simulink subsystem "SubsystemT"  (R2021a)
settings: Solver=VariableStepAuto  StartTime=0.0  StopTime=10.0  RelTol=1e-3
libraries: dspmathops x1, sharedtransform x1
settings Model: Creator=noraw  LastModifiedBy=noraw

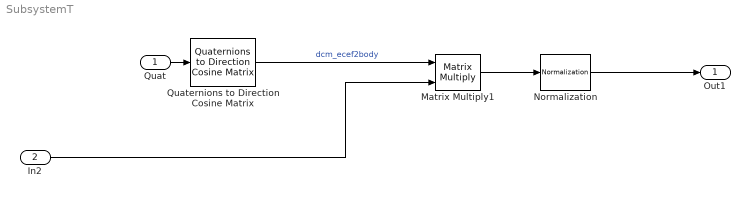
== system SubsystemT ==
  Quat : Inport
  In2 : Inport  Port=2
  Matrix Multiply1 : Product  Multiplication=Matrix(*)
  Normalization : dspmathops/Normalization  NormType=Squared 2-norm  Bias=1e-10  NormOver=Each column  Dimension=1  roundingMode=Floor  overflowMode=off  accumDataTypeStr=Inherit: Same as product output  accumLastDataTypeStr=Inherit: Same as product output  outputDataTypeStr=Inherit: Same as product output  outputMin=[]  outputMax=[]  outputLastDataTypeStr=Inherit: Same as product output
  Quaternions to Direction Cosine Matrix : sharedtransform/Quaternions to  Direction Cosine Matrix  aMode=aMode
      settings: SourceProductBaseCode=AE,PW,DR,MT,UV,VE
  Out1 : Outport
  wires:
  Matrix Multiply1/1 -> Normalization/1
  Quat/1 -> Quaternions to Direction Cosine Matrix/1
  Quaternions to Direction Cosine Matrix/1 -> Matrix Multiply1/1  "dcm_ecef2body"
  In2/1 -> Matrix Multiply1/2
  Normalization/1 -> Out1/1
